simulink model "dpt_model"  (R2023a)
settings: Solver=VariableStepAuto  StartTime=0.0  StopTime=10.0  RelTol=1e-3
values from neighbouring files (symbols this model uses):
  b = 0.001    [init.m]
  Cm = 1.3    [init.m]
  Cw = 3.15    [init.m]
  Jen = 7e-6    (= 7e-06)    [init.m]
  Lov = 0.013    [init.m]
  Lya = 0.0015    [init.m]
  Rya = 8    [init.m]
  Uupr = 5    [init.m]
settings Model: Creator=Алексей  LastModifiedBy=agalimov

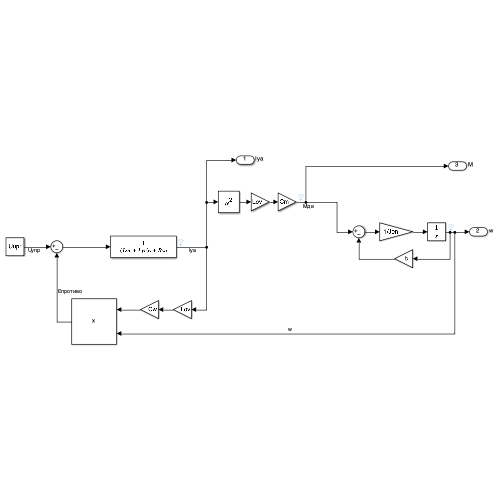
[thumbnail: Simulink's stored preview of the top-level diagram]
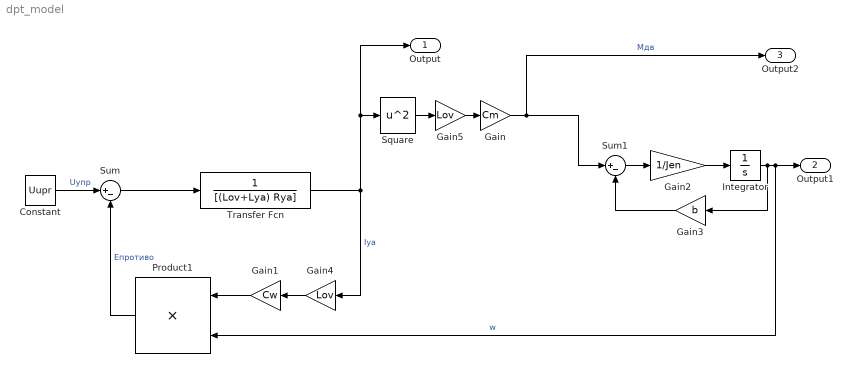
== system dpt_model ==
  Constant : Constant  Value=Uupr
  Gain : Gain  Gain=Cm
  Gain1 : Gain  Gain=Cw
  Gain2 : Gain  Gain=1/Jen
  Gain3 : Gain  Gain=b
  Gain4 : Gain  Gain=Lov
  Gain5 : Gain  Gain=Lov
  Integrator : Integrator
  Product1 : Product
  Square : Math  Operator=square
  Sum : Sum  Inputs=|+-
  Sum1 : Sum  Inputs=|+-
  Transfer Fcn : TransferFcn  Denominator=[(Lov+Lya) Rya]
  Output : Outport  SignalName=Iya
  Output1 : Outport  Port=2  SignalName=w
  Output2 : Outport  Port=3  SignalName=M
  wires:
  Constant/1 -> Sum/1  "Uупр"
  Sum/1 -> Transfer Fcn/1
  Transfer Fcn/1 -> Output/1, Square/1, Gain4/1  "Iya"
  Product1/1 -> Sum/2  "Епротиво"
  Integrator/1 -> Gain3/1, Output1/1, Product1/2  "w"
  Gain1/1 -> Product1/1
  Square/1 -> Gain5/1
  Gain/1 -> Sum1/1, Output2/1  "Мдв"
  Gain2/1 -> Integrator/1
  Gain4/1 -> Gain1/1
  Gain5/1 -> Gain/1
  Sum1/1 -> Gain2/1
  Gain3/1 -> Sum1/2
